simulink model "Iris_DeePC_Control_Linear"  (R2022a)
settings: Solver=VariableStepAuto  StartTime=0.0  StopTime=sim_time  RelTol=1e-3
values from neighbouring files (symbols this model uses):
  Ad = param.Ad_sys    [DeePC_main.m]    (also in collect_DeePC_data.m)
  Bd = param.Bd_sys    [DeePC_main.m]    (also in collect_DeePC_data.m)
  param = load_crazyflie_parameters()    [DeePC_main.m]
  start_time = 2    [DeePC_main.m]
undefined symbols (not defined in the file or in its folder): DeePC_param
libraries: Crazyflie_Library x2
settings Model: Creator=ezzat  LastModifiedBy=simao
settings SolverCC: AlgebraicLoopSolver=LineSearch
settings DataIOCC: ReturnWorkspaceOutputs=off
settings DebuggingCC: UnconnectedInputMsg=warning  UnconnectedOutputMsg=warning  UnconnectedLineMsg=warning  SFMachineParentedDataDiag=warning  ArithmeticOperatorsInVariantConditions=warning
settings SFSimCC: CustomCodeUndefinedFunction=UseInterfaceOnly

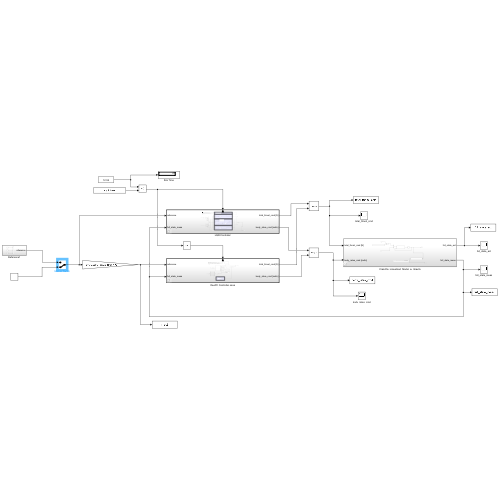
[thumbnail: Simulink's stored preview of the top-level diagram]
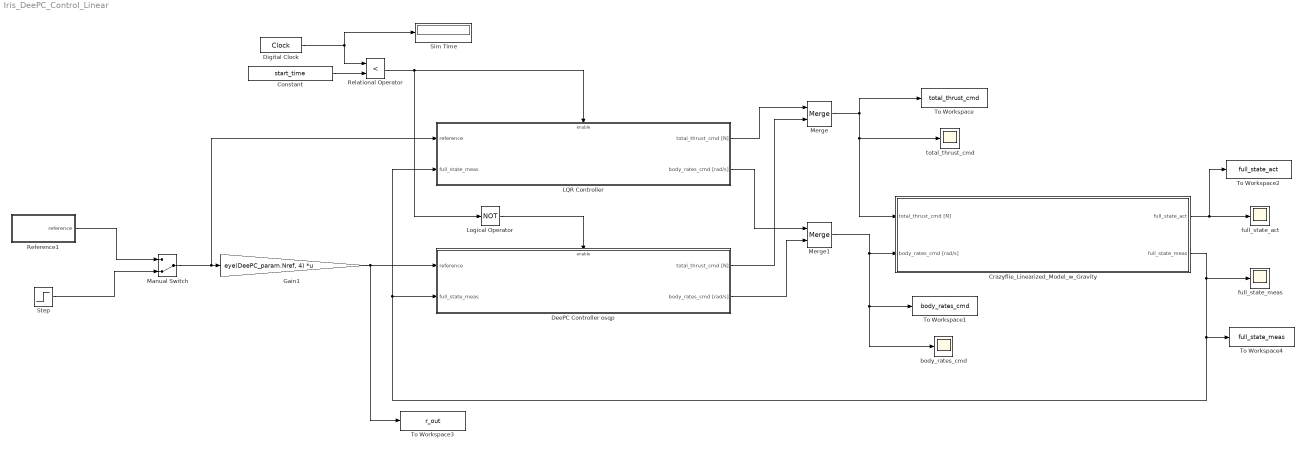
== system Iris_DeePC_Control_Linear ==
  Constant : Constant  Value=start_time
  Crazyflie_Linearized_Model_w_Gravity : Subsystem  AncestorBlock=Crazyflie_Library/Crazyflie_Linearized_Model_w_Gravity
  DeePC Controller osqp : Subsystem  AncestorBlock=Crazyflie_Library/DeePC_Controller_osqp
  Digital Clock : DigitalClock  SampleTime=param.sample_time_controller_outer
  Gain1 : Gain  Gain=eye(DeePC_param.Nref, 4)  Multiplication=Matrix(K*u)
  LQR Controller : Subsystem  AncestorBlock=Crazyflie_Library/LQR_Controller
  Logical Operator : Logic  Operator=NOT  AllPortsSameDT=off  OutDataTypeStr=boolean
  Manual Switch : ManualSwitch  CurrentSetting=0
  Merge : Merge
  Merge1 : Merge
  Reference1 : Subsystem
  Relational Operator : RelationalOperator  Operator=<  OutDataTypeStr=boolean  RndMeth=Simplest  InputSameDT=off
  Sim Time : Display
  Step : Step  Time=start_time  Before=[param.nrotor_initial_condition(1:3); param.nrotor_initial_condition(9)]  After=[param.nrotor_final_condition(1:3); param.nrotor_final_condition(9)]  SampleTime=0
  To Workspace : ToWorkspace  VariableName=total_thrust_cmd  SampleTime=param.sample_time_controller_outer
  To Workspace1 : ToWorkspace  VariableName=body_rates_cmd  SampleTime=param.sample_time_controller_outer
  To Workspace2 : ToWorkspace  VariableName=full_state_act  SampleTime=param.sample_time_controller_outer
  To Workspace3 : ToWorkspace  VariableName=r_out  SampleTime=param.sample_time_controller_outer
  To Workspace4 : ToWorkspace  VariableName=full_state_meas  SampleTime=param.sample_time_controller_outer
  body_rates_cmd : Scope
  full_state_act : Scope
  full_state_meas : Scope
  total_thrust_cmd : Scope
  wires:
  Crazyflie_Linearized_Model_w_Gravity/1(full_state_act) -> To Workspace2/1, full_state_act/1
  Crazyflie_Linearized_Model_w_Gravity/2(full_state_meas) -> To Workspace4/1, DeePC Controller osqp/2(full_state_meas), LQR Controller/2(full_state_meas), full_state_meas/1
  Digital Clock/1 -> Sim Time/1, Relational Operator/1
  Constant/1 -> Relational Operator/2
  DeePC Controller osqp/1(total_thrust_cmd [N]) -> Merge/2
  Merge/1 -> To Workspace/1, Crazyflie_Linearized_Model_w_Gravity/1(total_thrust_cmd [N]), total_thrust_cmd/1
  Merge1/1 -> Crazyflie_Linearized_Model_w_Gravity/2(body_rates_cmd [rad/s]), To Workspace1/1, body_rates_cmd/1
  DeePC Controller osqp/2(body_rates_cmd [rad/s]) -> Merge1/2
  LQR Controller/2(body_rates_cmd [rad/s]) -> Merge1/1
  Logical Operator/1 -> DeePC Controller osqp/Enable
  LQR Controller/1(total_thrust_cmd [N]) -> Merge/1
  Gain1/1 -> DeePC Controller osqp/1(reference), To Workspace3/1
  Relational Operator/1 -> Logical Operator/1, LQR Controller/Enable
  Step/1 -> Manual Switch/2
  Reference1/1(reference) -> Manual Switch/1
  Manual Switch/1 -> LQR Controller/1(reference), Gain1/1

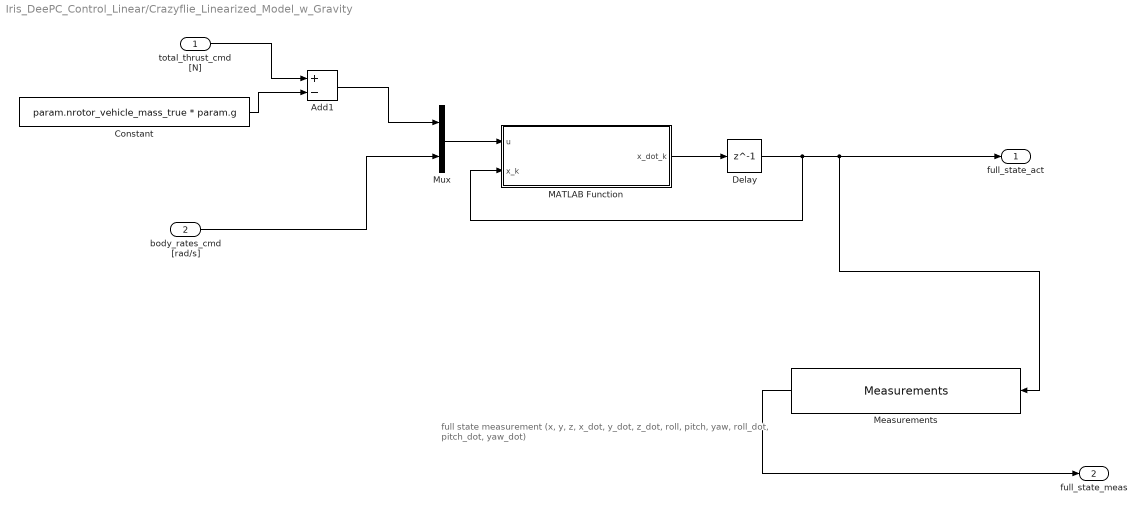
== system Iris_DeePC_Control_Linear/Crazyflie_Linearized_Model_w_Gravity ==
  note: full state measurement
      | (x, y, z, x_dot, y_dot, z_dot, roll, pitch, yaw, roll_dot, pitch_dot, yaw_dot)
  total_thrust_cmd [N] : Inport
  body_rates_cmd [rad/s] : Inport  Port=2
  Add1 : Sum  Inputs=+-
  Constant : Constant  Value=param.nrotor_vehicle_mass_true * param.g
  Delay : Delay  DelayLength=1  InitialCondition=param.nrotor_initial_condition(1:9)
  MATLAB Function : MATLAB Function  TreatAsAtomicUnit=on
  Measurements : Crazyflie_Library/Crazyflie_Linearized_Model_w_Gravity/Measurements  SystemSampleTime=-1  VariantActivationTime=update diagram  Latency=0  AutoFrameSizeCalculation=off
  Mux : Mux  Inputs=2
  full_state_act : Outport  VectorParamsAs1DForOutWhenUnconnected=off
  full_state_meas : Outport  Port=2  VectorParamsAs1DForOutWhenUnconnected=off
  wires:
  Delay/1 -> MATLAB Function/2(x_k), Measurements/1, full_state_act/1
  MATLAB Function/1(x_dot_k) -> Delay/1
  total_thrust_cmd [N]/1 -> Add1/1
  Add1/1 -> Mux/1
  Constant/1 -> Add1/2
  Mux/1 -> MATLAB Function/1(u)
  body_rates_cmd [rad/s]/1 -> Mux/2
  Measurements/1 -> full_state_meas/1

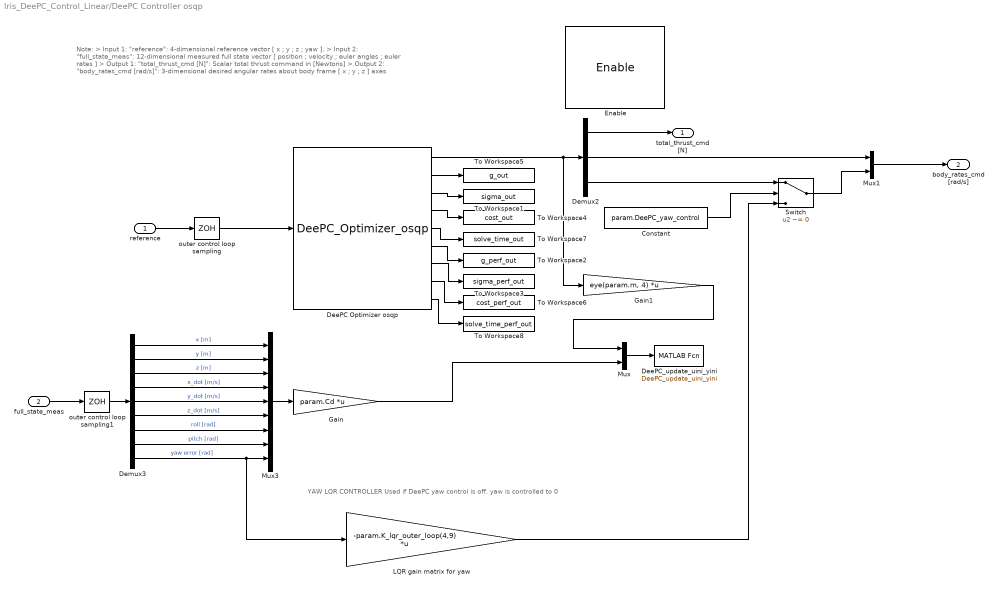
== system Iris_DeePC_Control_Linear/DeePC Controller osqp ==
  note: YAW LQR CONTROLLER
      | Used if DeePC yaw control is off. yaw is controlled to 0
  note: Note:
      | > Input 1: "reference": 4-dimensional reference vector [ x ; y ; z ; yaw ].
      | > Input 2: "full_state_meas": 12-dimensional measured full state vector [ position ; velocity ; euler angles ; euler rates ]
      | > Output 1: "total_thrust_cmd [N]": Scalar total thrust command in [Newtons]
      | > Output 2: "body_rates_cmd [rad/s]": 3-dimensional desired angular rates about body frame [ x ; y ; z ] axes
  reference : Inport
  full_state_meas : Inport  Port=2
  Enable : EnablePort
  Constant : Constant  Value=param.DeePC_yaw_control
  DeePC Optimizer osqp : Crazyflie_Library/DeePC_Optimizer_osqp  SystemSampleTime=-1  VariantActivationTime=update diagram  Latency=0  AutoFrameSizeCalculation=off
  DeePC_update_uini_yini : MATLABFcn  MATLABFcn=DeePC_update_uini_yini  OutputDimensions=0
  Demux2 : Demux  Outputs=[1 2 1]
  Demux3 : Demux  Outputs=9
  Gain : Gain  Gain=param.Cd  Multiplication=Matrix(K*u)
  Gain1 : Gain  Gain=eye(param.m, 4)  Multiplication=Matrix(K*u)
  LQR gain matrix for yaw : Gain  Gain=-param.K_lqr_outer_loop(4,9)  Multiplication=Matrix(K*u)
  Mux : Mux  Inputs=2
  Mux1 : Mux  Inputs=[2 1]
  Mux3 : Mux  Inputs=9
  Switch : Switch  Criteria=u2 ~= 0  SaturateOnIntegerOverflow=off  InputSameDT=off
  To Workspace1 : ToWorkspace  VariableName=sigma_out  SampleTime=-1
  To Workspace2 : ToWorkspace  VariableName=g_perf_out  SampleTime=-1
  To Workspace3 : ToWorkspace  VariableName=sigma_perf_out  SampleTime=-1
  To Workspace4 : ToWorkspace  VariableName=cost_out  SampleTime=-1
  To Workspace5 : ToWorkspace  VariableName=g_out  SampleTime=-1
  To Workspace6 : ToWorkspace  VariableName=cost_perf_out  SampleTime=-1
  To Workspace7 : ToWorkspace  VariableName=solve_time_out  SampleTime=-1
  To Workspace8 : ToWorkspace  VariableName=solve_time_perf_out  SampleTime=-1
  outer control loop sampling : ZeroOrderHold  SampleTime=param.sample_time_controller_outer
  outer control loop sampling1 : ZeroOrderHold  SampleTime=param.sample_time_controller_outer
  total_thrust_cmd [N] : Outport  VectorParamsAs1DForOutWhenUnconnected=off
  body_rates_cmd [rad/s] : Outport  Port=2  VectorParamsAs1DForOutWhenUnconnected=off
  wires:
  DeePC Optimizer osqp/7 -> To Workspace3/1
  DeePC Optimizer osqp/4 -> To Workspace4/1
  DeePC Optimizer osqp/3 -> To Workspace1/1
  DeePC Optimizer osqp/8 -> To Workspace6/1
  DeePC Optimizer osqp/6 -> To Workspace2/1
  DeePC Optimizer osqp/5 -> To Workspace7/1
  DeePC Optimizer osqp/9 -> To Workspace8/1
  DeePC Optimizer osqp/2 -> To Workspace5/1
  Gain1/1 -> Mux/1
  Constant/1 -> Switch/2
  Switch/1 -> Mux1/2
  Demux2/3 -> Switch/1
  Demux3/9 -> LQR gain matrix for yaw/1, Mux3/9  "yaw error [rad]"
  LQR gain matrix for yaw/1 -> Switch/3
  Mux1/1 -> body_rates_cmd [rad/s]/1
  Demux2/2 -> Mux1/1
  DeePC Optimizer osqp/1 -> Demux2/1, Gain1/1
  Gain/1 -> Mux/2
  Mux/1 -> DeePC_update_uini_yini/1
  outer control loop sampling/1 -> DeePC Optimizer osqp/1
  Demux2/1 -> total_thrust_cmd [N]/1
  Mux3/1 -> Gain/1
  outer control loop sampling1/1 -> Demux3/1
  reference/1 -> outer control loop sampling/1
  full_state_meas/1 -> outer control loop sampling1/1
  Demux3/5 -> Mux3/5  "y_dot [m/s]"
  Demux3/4 -> Mux3/4  "x_dot [m/s]"
  Demux3/7 -> Mux3/7  "roll [rad]"
  Demux3/8 -> Mux3/8  "pitch [rad]"
  Demux3/2 -> Mux3/2  "y [m]"
  Demux3/6 -> Mux3/6  "z_dot [m/s]"
  Demux3/3 -> Mux3/3  "z [m]"
  Demux3/1 -> Mux3/1  "x [m]"

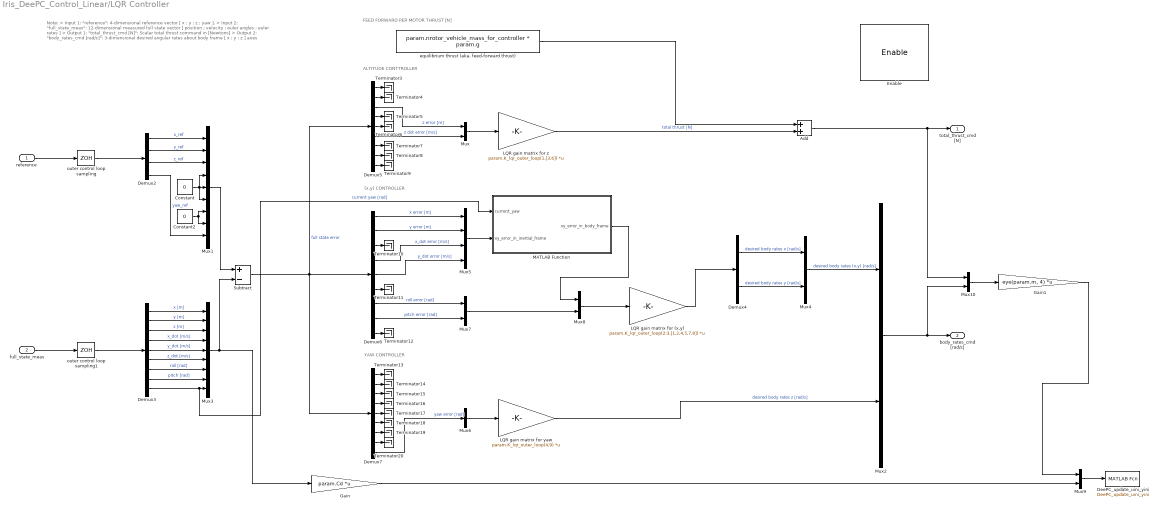
== system Iris_DeePC_Control_Linear/LQR Controller ==
  note: (x,y) CONTROLLER
  note: YAW CONTROLLER
  note: FEED FORWARD PER MOTOR THRUST [N]
  note: ALTITUDE CONTTROLLER
  note: Note:
      | > Input 1: "reference": 4-dimensional reference vector [ x ; y ; z ; yaw ].
      | > Input 2: "full_state_meas": 12-dimensional measured full state vector [ position ; velocity ; euler angles ; euler rates ]
      | > Output 1: "total_thrust_cmd [N]": Scalar total thrust command in [Newtons]
      | > Output 2: "body_rates_cmd [rad/s]": 3-dimensional desired angular rates about body frame [ x ; y ; z ] axes
  reference : Inport
  full_state_meas : Inport  Port=2
  Enable : EnablePort
  Add : Sum
  Constant : Constant  Value=0
  Constant2 : Constant  Value=0
  DeePC_update_uini_yini : MATLABFcn  MATLABFcn=DeePC_update_uini_yini  OutputDimensions=0
  Demux2 : Demux
  Demux{3,5..7} (4 alike) : Demux  Outputs=9
  Demux4 : Demux  Outputs=2
  Gain : Gain  Gain=param.Cd  Multiplication=Matrix(K*u)
  Gain1 : Gain  Gain=eye(param.m, 4)  Multiplication=Matrix(K*u)
  LQR gain matrix for (x,y) : Gain  Gain=param.K_lqr_outer_loop(2:3,[1,2,4,5,7,8])  Multiplication=Matrix(K*u)
  LQR gain matrix for yaw : Gain  Gain=param.K_lqr_outer_loop(4,9)  Multiplication=Matrix(K*u)
  LQR gain matrix for z : Gain  Gain=param.K_lqr_outer_loop(1,[3,6])  Multiplication=Matrix(K*u)
  MATLAB Function : MATLAB Function  TreatAsAtomicUnit=on
  Mux{,2,4,7..10} (7 alike) : Mux  Inputs=2
  Mux1 : Mux  Inputs=9
  Mux3 : Mux  Inputs=9
  Mux5 : Mux
  Mux6 : Mux  Inputs=1
  Subtract : Sum  Inputs=+-
  Terminator{3..20} (18 alike) : Terminator
  equilibrium thrust (aka. feed-forward thrust) : Constant  Value=param.nrotor_vehicle_mass_for_controller * param.g
  outer control loop sampling : ZeroOrderHold  SampleTime=param.sample_time_controller_outer
  outer control loop sampling1 : ZeroOrderHold  SampleTime=param.sample_time_controller_outer
  total_thrust_cmd [N] : Outport  VectorParamsAs1DForOutWhenUnconnected=off
  body_rates_cmd [rad/s] : Outport  Port=2  VectorParamsAs1DForOutWhenUnconnected=off
  wires:
  Mux10/1 -> Gain1/1
  Gain1/1 -> Mux9/1
  Gain/1 -> Mux9/2
  Mux3/1 -> Subtract/2, Gain/1
  Mux2/1 -> body_rates_cmd [rad/s]/1, Mux10/2
  Add/1 -> Mux10/1, total_thrust_cmd [N]/1
  Mux9/1 -> DeePC_update_uini_yini/1
  equilibrium thrust (aka. feed-forward thrust)/1 -> Add/1
  Demux7/4 -> Terminator16/1
  Demux5/4 -> Terminator5/1
  Demux7/9 -> Mux6/1  "yaw error [rad]"
  LQR gain matrix for z/1 -> Add/2  "total thrust [N]"
  Demux7/5 -> Terminator17/1
  Demux7/6 -> Terminator18/1
  Demux2/1 -> Mux1/1  "x_ref"
  Mux7/1 -> Mux8/2
  Demux3/1 -> Mux3/1  "x [m]"
  Demux7/3 -> Terminator15/1
  Mux4/1 -> Mux2/1  "desired body rates (x,y) [rad/s]"
  Demux3/3 -> Mux3/3  "z [m]"
  Demux3/6 -> Mux3/6  "z_dot [m/s]"
  Demux6/5 -> Mux5/4  "y_dot error [m/s]"
  Constant/1 -> Mux1/5, Mux1/4, Mux1/6
  Constant2/1 -> Mux1/7, Mux1/8
  Demux6/6 -> Terminator11/1
  Demux3/2 -> Mux3/2  "y [m]"
  Demux2/4 -> Mux1/9  "yaw_ref"
  Demux3/8 -> Mux3/8  "pitch [rad]"
  Demux6/4 -> Mux5/3  "x_dot error [m/s]"
  Demux3/9 -> MATLAB Function/1(current_yaw), Mux3/9  "current yaw [rad]"
  Demux3/7 -> Mux3/7  "roll [rad]"
  Demux2/2 -> Mux1/2  "y_ref"
  Demux5/6 -> Mux/2  "z dot error [m/s]"
  Subtract/1 -> Demux6/1, Demux5/1, Demux7/1  "full state error"
  Demux4/2 -> Mux4/2  "desired body rates y [rad/s]"
  LQR gain matrix for yaw/1 -> Mux2/2  "desired body rates z [rad/s]"
  Demux7/2 -> Terminator14/1
  Demux6/9 -> Terminator12/1
  Demux5/8 -> Terminator8/1
  Demux6/2 -> Mux5/2  "y error [m]"
  Demux6/8 -> Mux7/2  "pitch error [rad]"
  Demux3/4 -> Mux3/4  "x_dot [m/s]"
  Demux2/3 -> Mux1/3  "z_ref"
  Mux/1 -> LQR gain matrix for z/1
  Demux6/7 -> Mux7/1  "roll error [rad]"
  Demux7/1 -> Terminator13/1
  Demux5/3 -> Mux/1  "z error [m]"
  Demux7/8 -> Terminator20/1
  Mux5/1 -> MATLAB Function/2(xy_error_in_inertial_frame)
  Demux5/9 -> Terminator9/1
  Demux6/3 -> Terminator10/1
  Mux6/1 -> LQR gain matrix for yaw/1
  Demux5/2 -> Terminator4/1
  Demux6/1 -> Mux5/1  "x error [m]"
  MATLAB Function/1(xy_error_in_body_frame) -> Mux8/1
  Demux7/7 -> Terminator19/1
  Mux1/1 -> Subtract/1
  Mux8/1 -> LQR gain matrix for (x,y)/1
  Demux5/7 -> Terminator7/1
  LQR gain matrix for (x,y)/1 -> Demux4/1
  Demux4/1 -> Mux4/1  "desired body rates x [rad/s]"
  Demux3/5 -> Mux3/5  "y_dot [m/s]"
  Demux5/5 -> Terminator6/1
  Demux5/1 -> Terminator3/1
  full_state_meas/1 -> outer control loop sampling1/1
  outer control loop sampling/1 -> Demux2/1
  reference/1 -> outer control loop sampling/1
  outer control loop sampling1/1 -> Demux3/1

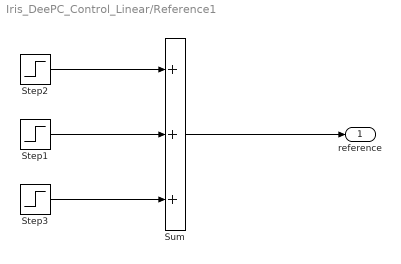
== system Iris_DeePC_Control_Linear/Reference1 ==
  Step1 : Step  Time=start_time+20  Before=[0;0;0;0]  After=[-1;-1;1;0]  SampleTime=0
  Step2 : Step  Time=start_time  Before=[param.nrotor_initial_condition(1:3); param.nrotor_initial_condition(9)]  After=[param.nrotor_final_condition(1:3); param.nrotor_final_condition(9)]  SampleTime=0
  Step3 : Step  Time=start_time+40  Before=[0;0;0;0]  After=[1;1;-1;0]  SampleTime=0
  Sum : Sum  Inputs=+++
  reference : Outport
  wires:
  Sum/1 -> reference/1
  Step2/1 -> Sum/1
  Step1/1 -> Sum/2
  Step3/1 -> Sum/3

== matlab function Iris_DeePC_Control_Linear/Crazyflie_Linearized_Model_w_Gravity/MATLAB Function ==
  data: u input; x_dot_k output; x_k input; Ad parameter; Bd parameter
function x_dot_k = fcn(u,x_k, Ad, Bd)

x_dot_k = zeros(9,1);

x_dot_k = Ad*x_k + Bd*u;

== matlab function Iris_DeePC_Control_Linear/LQR Controller/MATLAB Function ==
  data: current_yaw input; xy_error_in_inertial_frame input; xy_error_in_body_frame output
function xy_error_in_body_frame = rotate_xy_intertial_to_body( current_yaw , xy_error_in_inertial_frame )
% ----------------------------------------------------------------------- %
% DESCRIPTION:
% This function rotates an (x,y) coordainte and (x_dot,y_dot) velocity
% vector from the interial frame into (approximately) the body frame. The
% approximate is because the rotation into the body frame is only based on
% the current yaw of the vehicle and assumes that roll and pitch are zero.
%
%
% INPUT ARGUMENTS:
% current_yaw
% > The intrinsic Euler yaw angle, in radians
%
% xy_error_in_inertial_frame [m;m;m/s;m/s]
% > The measurement of (x,y) position and velocities in the inertial frame
%
%
% RETURN ARGUMENTS:
% xy_error_in_body_frame
% > The measurement of (x,y) position and velocities rotated into the body
%   frame
%
%
% ----------------------------------------------------------------------- %


% Extract the inertial position and velocities
x_I      =  xy_error_in_inertial_frame(1);
y_I      =  xy_error_in_inertial_frame(2);
xdot_I   =  xy_error_in_inertial_frame(3);
ydot_I   =  xy_error_in_inertial_frame(4);

% Save some computation
cosYaw = cos(current_yaw);
sinYaw = sin(current_yaw);

% Initialise the return variable "xy_error_in_body_frame" to zeros
% > This can be required so that Simulink knows the expected size
xy_error_in_body_frame = zeros(4,1);


% Rotate the inertial POSITIONS into the body frame
% > For computing x in the body frame
xy_error_in_body_frame(1,1) =  x_I * cosYaw + y_I * sinYaw;
% > For computing y in the body frame
xy_error_in_body_frame(2,1) =  y_I * cosYaw - x_I * sinYaw;


% Rotate the inertial VELOCITIES into the body frame
% > For computing xdot in the body frame
xy_error_in_body_frame(3,1) =  xdot_I * cosYaw + ydot_I * sinYaw;
% > For computing ydot in the body frame
xy_error_in_body_frame(4,1) =  ydot_I * cosYaw - xdot_I * sinYaw;
